simulink model "sim_carroponte_CL_students"  (R2025b)
settings: Solver=FixedStepAuto  StartTime=0.0  StopTime=t(end)  FixedStep=mean(diff(t))  RelTol=1e-3
values from neighbouring files (symbols this model uses):
  l = 0.229    [Cerca_Poli_R.m]    (also in Estrai_G.m; Progetto_Regolatore.m; carroponte_inizializzazione_solution.m)
  R = K*(s^2 + 0.5803*s + 45)/((s + p1)*(s + p2))    [Cerca_Poli_R.m]    (also in Progetto_Regolatore.m = K*(s^2 + 0.5803*s + 45)/((s + p1_best)*(s + p2_best)); carroponte_inizializzazione_solution.m = 35*(s^2 + 0.5803*s + 45)/((s + p1_best)*(s + p2_best)))
  x0 = [0 0*pi/180 0 0]'    [Progetto_Regolatore.m]    (also in carroponte_inizializzazione_solution.m)
settings Model: Creator=Giulio  LastModifiedBy=anton
settings SolverCC: AlgebraicLoopSolver=TrustRegion
settings DataIOCC: ReturnWorkspaceOutputs=off
settings DebuggingCC: UnconnectedInputMsg=warning  UnconnectedOutputMsg=warning  UnconnectedLineMsg=warning  ArithmeticOperatorsInVariantConditions=warning
settings ModelReferenceCC: EnableRefExpFcnMdlSchedulingChecks=on
settings SFSimCC: SimUseLocalCustomCode=off  CustomCodeUndefinedFunction=UseInterfaceOnly
settings RTWCC: RTWUseLocalCustomCode=off  GPUComputeCapability=3.5
settings CodeAppCC: StateflowObjectComments=on

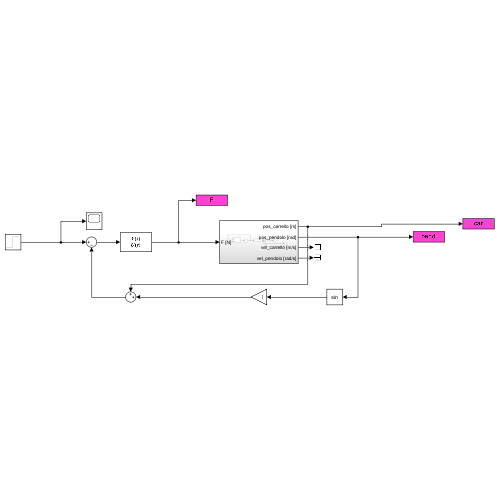
[thumbnail: Simulink's stored preview of the top-level diagram]
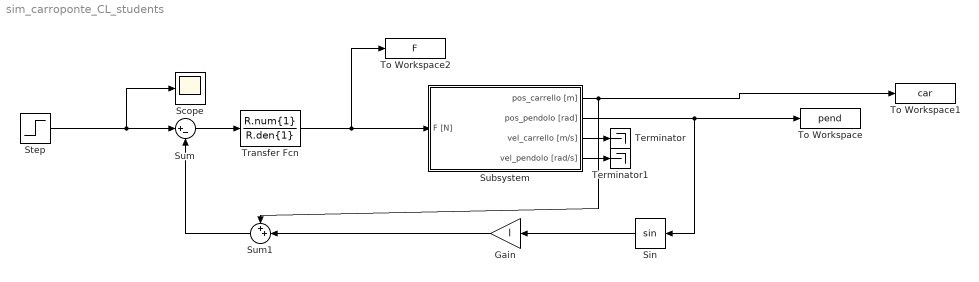
== system sim_carroponte_CL_students ==
  Gain : Gain  Gain=l
  Scope : Scope
      settings: ActiveDisplayYMinimum=-0.25  ActiveDisplayYMaximum=2.25
  Sin : Trigonometry
  Step : Step  Time=0  After=0.66  SampleTime=0
  Subsystem : Subsystem
  Sum : Sum  Inputs=|+-
  Sum1 : Sum  Inputs=++|
  Terminator : Terminator
  Terminator1 : Terminator
  To Workspace : ToWorkspace  VariableName=pend  SampleTime=-1
  To Workspace1 : ToWorkspace  VariableName=car  SampleTime=-1
  To Workspace2 : ToWorkspace  VariableName=F  SampleTime=-1
  Transfer Fcn : TransferFcn  Numerator=R.num{1}  Denominator=R.den{1}
  wires:
  Step/1 -> Scope/1, Sum/1
  Subsystem/1(pos_carrello [m]) -> To Workspace1/1, Sum1/1
  Subsystem/3(vel_carrello [m/s]) -> Terminator/1
  Subsystem/4(vel_pendolo [rad/s]) -> Terminator1/1
  Subsystem/2(pos_pendolo [rad]) -> To Workspace/1, Sin/1
  Sum/1 -> Transfer Fcn/1
  Transfer Fcn/1 -> To Workspace2/1, Subsystem/1(F [N])
  Gain/1 -> Sum1/2
  Sin/1 -> Gain/1
  Sum1/1 -> Sum/2

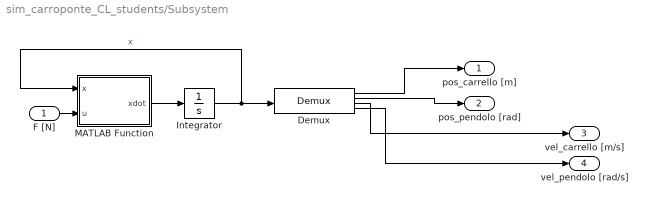
== system sim_carroponte_CL_students/Subsystem ==
  F [N] : Inport
  Demux : Demux
      settings: DisplayOption=none
  Integrator : Integrator  InitialCondition=x0
  MATLAB Function : MATLAB Function  TreatAsAtomicUnit=on
  pos_carrello [m] : Outport
  pos_pendolo [rad] : Outport  Port=2
  vel_carrello [m/s] : Outport  Port=3
  vel_pendolo [rad/s] : Outport  Port=4
  wires:
  Demux/1 -> pos_carrello [m]/1
  F [N]/1 -> MATLAB Function/2(u)
  Demux/3 -> vel_carrello [m/s]/1
  Demux/4 -> vel_pendolo [rad/s]/1
  Demux/2 -> pos_pendolo [rad]/1
  MATLAB Function/1(xdot) -> Integrator/1
  Integrator/1 -> MATLAB Function/1(x), Demux/1  "x"

== matlab function sim_carroponte_CL_students/Subsystem/MATLAB Function ==
  data: x input; u input; xdot output
function xdot = fcn(x,u)
%CARRO Summary of this function goes here
%   x = [x t xd td]

%% Parametri
l       = 0.229;
M       = 0.57;
m       = 0.119;
mtot    = M + m;

J       = 4.458e-4;
Jtot    = m*l^2 + J;

cm      = 3;            % Forza attrito massa
cp      = 1e-5;         % Forza attrito pendolo 

g = 9.81;

%% Stato
x1 = x(1);      % x
x2 = x(2);      % teta
x3 = x(3);      % x dot
x4 = x(4);      % teta dot

%% Equazioni nonlineari
xdot1 = x3;
xdot2 = x4;
xdot3 = (-Jtot*cm*x3   +   m*l*cp*cos(x2)*x4                  +   m*l*Jtot*sin(x2)*x4^2   +   m^2*l^2*g*sin(x2)*cos(x2)   +   Jtot*u)         /(Jtot*mtot - m^2*l^2*cos(x2)^2);
xdot4 = (-mtot*cp*x4   -   m^2*l^2*sin(x2)*cos(x2)*x4^2       +   cm*m*l*cos(x2)*x3       -   mtot*m*l*g*sin(x2)          -   m*l*cos(x2)*u)  /(Jtot*mtot - m^2*l^2*cos(x2)^2);

%% Uscita
xdot = [xdot1;
        xdot2;
        xdot3;
        xdot4];

end
